simulink model "feedback"  (R2022a)
settings: Solver=VariableStepAuto  StartTime=0.0  StopTime=50  RelTol=1e-3
values from neighbouring files (symbols this model uses):
  A = [0 0 0 1 0 0 ... (first row only)    [main.m]
  B = [0 0 ... (first row only)    [main.m]
  C = [1 0 0 0 0 0 ... (first row only)    [main.m]
  klqr2 = real(inv(R)*B'*P2)    [main.m]
  x0 = [0.2 -0.1 0.15 -1 0.8 0]'    [main.m]
settings Model: Creator=qidon  LastModifiedBy=dzsgy

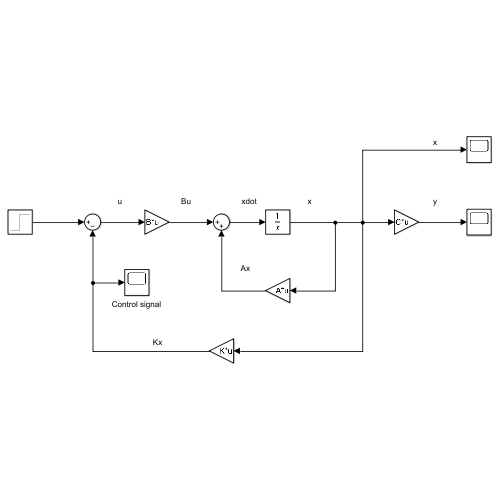
[thumbnail: Simulink's stored preview of the top-level diagram]
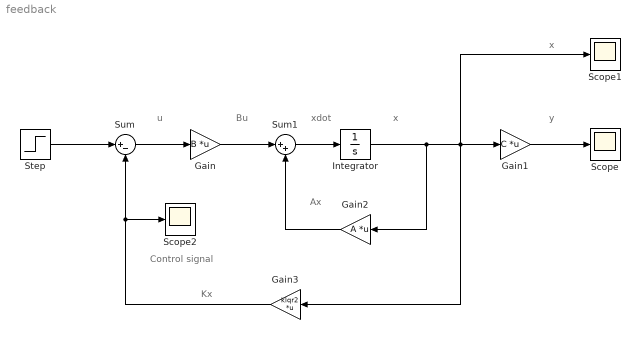
== system feedback ==
  note: Kx
  note: x
  note: y
  note: Ax
  note: Bu
  note: x
  note: u
  note: Control signal
  note: xdot
  Gain : Gain  Gain=B  Multiplication=Matrix(K*u)
  Gain1 : Gain  Gain=C  Multiplication=Matrix(K*u)
  Gain2 : Gain  Gain=A  Multiplication=Matrix(K*u)
  Gain3 : Gain  Gain=klqr2  Multiplication=Matrix(K*u)
  Integrator : Integrator  InitialCondition=x0
  Scope : Scope
  Scope1 : Scope
  Scope2 : Scope
  Step : Step  Time=0  After=0  SampleTime=0
  Sum : Sum  Inputs=|+-
  Sum1 : Sum  Inputs=|++
  wires:
  Gain3/1 -> Scope2/1, Sum/2
  Sum/1 -> Gain/1
  Gain/1 -> Sum1/1
  Sum1/1 -> Integrator/1
  Gain2/1 -> Sum1/2
  Integrator/1 -> Gain2/1, Scope1/1, Gain3/1, Gain1/1
  Gain1/1 -> Scope/1
  Step/1 -> Sum/1
